simulink model "Observador_estados_discreto_plantilla_con_regulador"  (R2016a)
settings: Solver=VariableStepAuto  StartTime=0.0  StopTime=10.0  RelTol=1e-3
values from neighbouring files (symbols this model uses):
  h = place(A_dis',C_dis',Po)'    [Regulador_seguidor_observador_codigo.m]
  k = place(A_dis,B_dis,Pol_des_dis)    [Regulador_seguidor_observador_codigo.m]
  tm = 0.1    [Regulador_seguidor_observador_codigo.m]
undefined symbols (not defined in the file or in its folder): A_dis, B_dis, C_dis
settings Model: Creator=Daniel  LastModifiedBy=Daniel

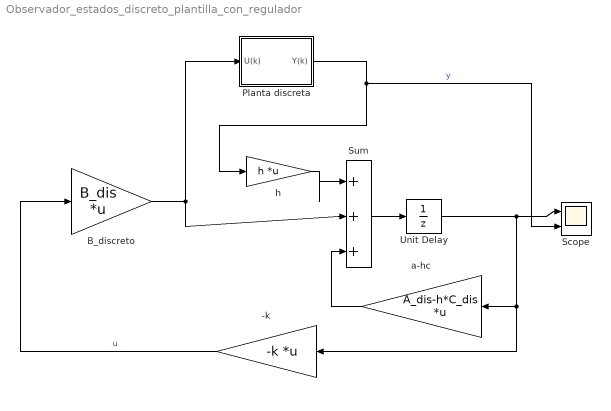
== system Observador_estados_discreto_plantilla_con_regulador ==
  -k : Gain  Gain=-k  Multiplication=Matrix(K*u) (u vector)
  B_discreto : Gain  Gain=B_dis  Multiplication=Matrix(K*u) (u vector)
  Planta discreta : Subsystem
  Scope : Scope  NumInputPorts=2
  Sum : Sum  Inputs=|+++
  Unit Delay : UnitDelay  SampleTime=tm
  a-hc : Gain  Gain=A_dis-h*C_dis  Multiplication=Matrix(K*u) (u vector)
  h : Gain  Gain=h  Multiplication=Matrix(K*u) (u vector)
  wires:
  Sum/1 -> Unit Delay/1
  a-hc/1 -> Sum/3
  h/1 -> Sum/1
  Planta discreta/1(Y(k)) -> Scope/2, h/1  "y"
  -k/1 -> B_discreto/1  "u"
  Unit Delay/1 -> Scope/1, -k/1, a-hc/1
  B_discreto/1 -> Planta discreta/1(U(k)), Sum/2

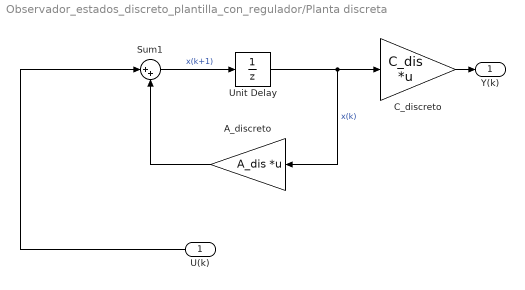
== system Observador_estados_discreto_plantilla_con_regulador/Planta discreta ==
  U(k) : Inport
  A_discreto : Gain  Gain=A_dis  Multiplication=Matrix(K*u) (u vector)
  C_discreto : Gain  Gain=C_dis  Multiplication=Matrix(K*u) (u vector)
  Sum1 : Sum  Inputs=|++
  Unit Delay : UnitDelay  InitialCondition=[1;1]  SampleTime=tm
  Y(k) : Outport
  wires:
  Unit Delay/1 -> A_discreto/1, C_discreto/1  "x(k)"
  A_discreto/1 -> Sum1/2
  Sum1/1 -> Unit Delay/1  "x(k+1)"
  C_discreto/1 -> Y(k)/1
  U(k)/1 -> Sum1/1
